simulink model "elec522_sysgen_block_LAB3"  (Simulink 8.9)
settings: Solver=VariableStepAuto  StartTime=0.0  StopTime=30  RelTol=1e-3
libraries: xbsIndex_r4 x41
settings Model: Creator=rl59  LastModifiedBy=rl59
settings DataIOCC: LimitDataPoints=off  SaveFormat=Dataset  SignalLoggingSaveFormat=Dataset
settings OptimizationCC: LifeSpan=auto
settings DebuggingCC: UnderspecifiedInitializationDetection=Simplified  MergeDetectMultiDrivingBlocksExec=error  FcnCallInpInsideContextMsg=error  StateNameClashWarn=none  SFUnexpectedBacktrackingDiag=error  SFNoUnconditionalDefaultTransitionDiag=error  SFExecutionAtInitializationDiag=warning
settings HardwareCC: ProdBitPerPointer=64  ProdBitPerSizeT=64  ProdBitPerPtrDiffT=64  ProdLargestAtomicFloat=Float  ProdIntDivRoundTo=Zero  ProdEndianess=LittleEndian  ProdWordSize=64  ProdHWDeviceType=Intel->x86-64 (Windows64)
settings ModelReferenceCC: PropagateSignalLabelsOutOfModel=on
settings GRTTargetCC: TargetLangStandard=C99 (ISO)  GeneratePreprocessorConditionals=Use local settings  CombineOutputUpdateFcns=on  GRTInterface=off
settings ConfigComp: CovMetricSettings=dwe  CovHtmlReporting=off  CovSaveCumulativeToWorkspaceVar=off  CovSaveSingleToWorkspaceVar=off  CovExternalEMLEnable=on

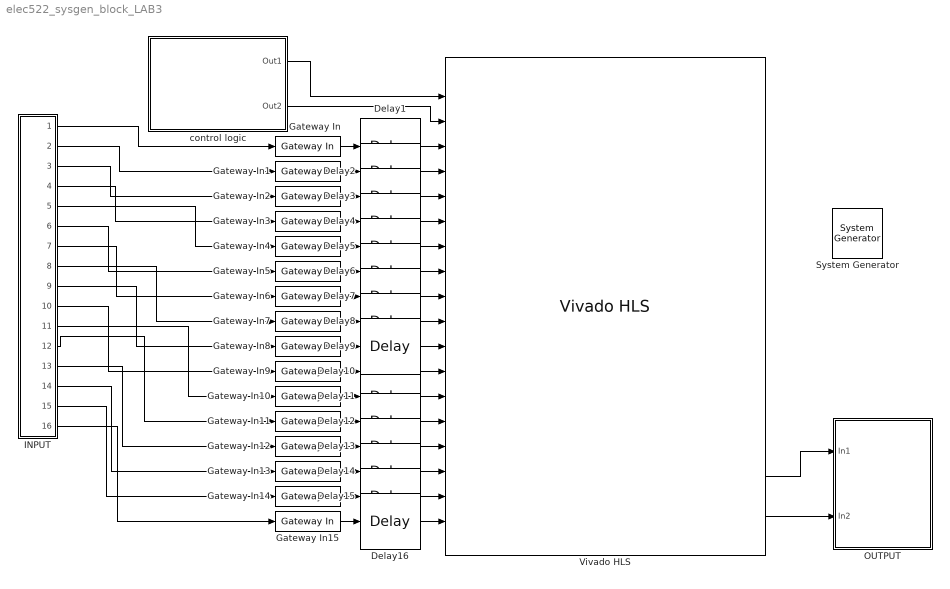
== system elec522_sysgen_block_LAB3 ==
  " System Generator" : xbsIndex_r4/ System Generator  Tag=genX  xilinxfamily=kintex7  part=xc7k325t  speed=-3  package=fbg676  synthesis_tool=Vivado  clock_wrapper=Clock Enables  directory=./netlist  proj_type=Vivado  Synth_file=Vivado Synthesis Defaults  Impl_file=Vivado Implementation Defaults  testbench=off  simulink_period=1  sysclk_period=10  dcm_input_clock_period=10  incr_netlist=off  trim_vbits=Everywhere in SubSystem  dbl_ovrd=According to Block Masks  core_generation=According to Block Masks  run_coregen=off  deprecated_control=off  eval_field=0  block_type=sysgen
  Delay{1..16} (16 alike) : xbsIndex_r4/Delay  rst=off  infoeditControl=Selection of Reset will increase slice count due to use of real FFs and instead of SRLs  en=off  latency=4  reg_retiming=off  dbl_ovrd=off  block_type=delay
  Gateway In{,1..15} (16 alike) : xbsIndex_r4/Gateway In  gui_display_data_type=Fixed-point  arith_type="Signed  (2's comp)"  n_bits=16  bin_pt=0  preci_type=Single  exp_width=8  frac_width=24  rows=1  columns=1  quantization="Round  (unbiased: +/- Inf)"  overflow=Saturate  period=1  UseAsADC=off  ADCChannel='1'  interface=None  automatic_assignment=on  address_offset=hex2dec('00')  intf_name=''  intf_description=''  default_value=0  timing_constraint=None  locs_specified=off  LOCs={}  io_standard={}  inherit_from_input=off  hdl_port=on  dbl_ovrd=off  block_type=gatewayin
  INPUT : Subsystem
  OUTPUT : Subsystem
  Vivado HLS : xbsIndex_r4/Vivado HLS  anytable='C:/Users/rl59/Desktop/ELEC522_project3_RAN.LU_WEIXU.PAN/ELEC522_project3_RAN.LU_WEIXU.PAN/ELEC522_project3/solution6'  fast_sim=off  display_datatype=on  rate_propagation_method=Simulink system period  model_file_path=''  latency=1  block_type=hls
      settings: infoedit=This block allows including C,C++ and SystemC source files in System Generator for DSP designs.
  "control logic " : Subsystem
  wires:
  Gateway In/1 -> Delay1/1
  Delay1/1 -> Vivado HLS/3
  Gateway In1/1 -> Delay2/1
  Delay2/1 -> Vivado HLS/4
  Gateway In2/1 -> Delay3/1
  Delay3/1 -> Vivado HLS/5
  Gateway In3/1 -> Delay4/1
  Delay4/1 -> Vivado HLS/6
  Gateway In4/1 -> Delay5/1
  Delay5/1 -> Vivado HLS/7
  Gateway In5/1 -> Delay6/1
  Delay6/1 -> Vivado HLS/8
  Gateway In6/1 -> Delay7/1
  Delay7/1 -> Vivado HLS/9
  Gateway In7/1 -> Delay8/1
  Delay8/1 -> Vivado HLS/10
  Gateway In8/1 -> Delay9/1
  Delay9/1 -> Vivado HLS/11
  Gateway In9/1 -> Delay10/1
  Delay10/1 -> Vivado HLS/12
  Gateway In10/1 -> Delay11/1
  Delay11/1 -> Vivado HLS/13
  Gateway In11/1 -> Delay12/1
  Delay12/1 -> Vivado HLS/14
  Gateway In12/1 -> Delay13/1
  Delay13/1 -> Vivado HLS/15
  Gateway In13/1 -> Delay14/1
  Delay14/1 -> Vivado HLS/16
  Gateway In14/1 -> Delay15/1
  Delay15/1 -> Vivado HLS/17
  Gateway In15/1 -> Delay16/1
  Delay16/1 -> Vivado HLS/18
  INPUT/1(Out1) -> Gateway In/1
  INPUT/2(Out2) -> Gateway In1/1
  INPUT/3(Out3) -> Gateway In2/1
  INPUT/4(Out4) -> Gateway In3/1
  INPUT/5(Out5) -> Gateway In4/1
  INPUT/6(Out6) -> Gateway In5/1
  INPUT/7(Out7) -> Gateway In6/1
  INPUT/8(Out8) -> Gateway In7/1
  INPUT/9(Out9) -> Gateway In8/1
  INPUT/10(Out10) -> Gateway In9/1
  INPUT/11(Out11) -> Gateway In10/1
  INPUT/12(Out12) -> Gateway In11/1
  INPUT/13(Out13) -> Gateway In12/1
  INPUT/14(Out14) -> Gateway In13/1
  INPUT/15(Out15) -> Gateway In14/1
  INPUT/16(Out16) -> Gateway In15/1
  Vivado HLS/39 -> OUTPUT/1(In1)
  Vivado HLS/43 -> OUTPUT/2(In2)
  "control logic "/1(Out1) -> Vivado HLS/1
  "control logic "/2(Out2) -> Vivado HLS/2

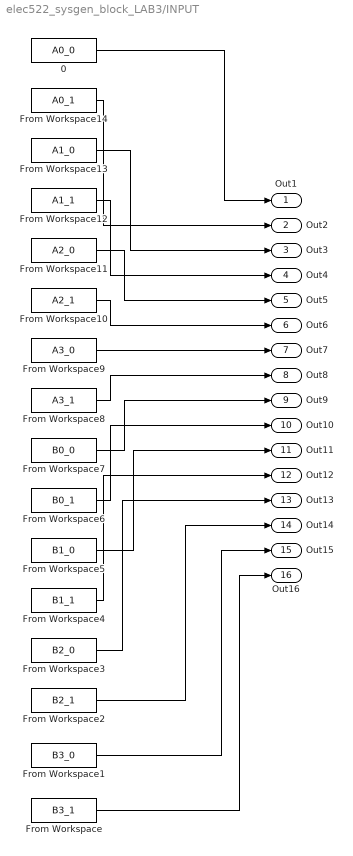
== system elec522_sysgen_block_LAB3/INPUT ==
  0 : FromWorkspace  VariableName=A0_0  SampleTime=1
  From Workspace : FromWorkspace  VariableName=B3_1  SampleTime=1
  From Workspace1 : FromWorkspace  VariableName=B3_0  SampleTime=1
  From Workspace10 : FromWorkspace  VariableName=A2_1  SampleTime=1
  From Workspace11 : FromWorkspace  VariableName=A2_0  SampleTime=1
  From Workspace12 : FromWorkspace  VariableName=A1_1  SampleTime=1
  From Workspace13 : FromWorkspace  VariableName=A1_0  SampleTime=1
  From Workspace14 : FromWorkspace  VariableName=A0_1  SampleTime=1
  From Workspace2 : FromWorkspace  VariableName=B2_1  SampleTime=1
  From Workspace3 : FromWorkspace  VariableName=B2_0  SampleTime=1
  From Workspace4 : FromWorkspace  VariableName=B1_1  SampleTime=1
  From Workspace5 : FromWorkspace  VariableName=B1_0  SampleTime=1
  From Workspace6 : FromWorkspace  VariableName=B0_1  SampleTime=1
  From Workspace7 : FromWorkspace  VariableName=B0_0  SampleTime=1
  From Workspace8 : FromWorkspace  VariableName=A3_1  SampleTime=1
  From Workspace9 : FromWorkspace  VariableName=A3_0  SampleTime=1
  Out1 : Outport
  Out2 : Outport  Port=2
  Out3 : Outport  Port=3
  Out4 : Outport  Port=4
  Out5 : Outport  Port=5
  Out6 : Outport  Port=6
  Out7 : Outport  Port=7
  Out8 : Outport  Port=8
  Out9 : Outport  Port=9
  Out10 : Outport  Port=10
  Out11 : Outport  Port=11
  Out12 : Outport  Port=12
  Out13 : Outport  Port=13
  Out14 : Outport  Port=14
  Out15 : Outport  Port=15
  Out16 : Outport  Port=16
  wires:
  From Workspace3/1 -> Out13/1
  From Workspace2/1 -> Out14/1
  From Workspace13/1 -> Out3/1
  From Workspace7/1 -> Out9/1
  From Workspace5/1 -> Out11/1
  From Workspace1/1 -> Out15/1
  From Workspace14/1 -> Out2/1
  From Workspace4/1 -> Out12/1
  From Workspace10/1 -> Out6/1
  From Workspace11/1 -> Out5/1
  0/1 -> Out1/1
  From Workspace6/1 -> Out10/1
  From Workspace12/1 -> Out4/1
  From Workspace/1 -> Out16/1
  From Workspace9/1 -> Out7/1
  From Workspace8/1 -> Out8/1

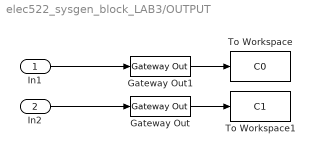
== system elec522_sysgen_block_LAB3/OUTPUT ==
  In1 : Inport
  In2 : Inport  Port=2
  Gateway Out : xbsIndex_r4/Gateway Out  inherit_from_input=off  hdl_port=on  rows=1  columns=1  UseAsDAC=off  DACChannel='1'  interface=None  automatic_assignment=on  address_offset=hex2dec('00')  intf_name=''  intf_description=''  timing_constraint=None  locs_specified=off  LOCs={}  io_standard={}  block_type=gatewayout
  Gateway Out1 : xbsIndex_r4/Gateway Out  inherit_from_input=off  hdl_port=on  rows=1  columns=1  UseAsDAC=off  DACChannel='1'  interface=None  automatic_assignment=on  address_offset=hex2dec('00')  intf_name=''  intf_description=''  timing_constraint=None  locs_specified=off  LOCs={}  io_standard={}  block_type=gatewayout
  To Workspace : ToWorkspace  VariableName=C0  SampleTime=-1
  To Workspace1 : ToWorkspace  VariableName=C1  SampleTime=-1
  wires:
  In2/1 -> Gateway Out/1
  In1/1 -> Gateway Out1/1
  Gateway Out/1 -> To Workspace1/1
  Gateway Out1/1 -> To Workspace/1

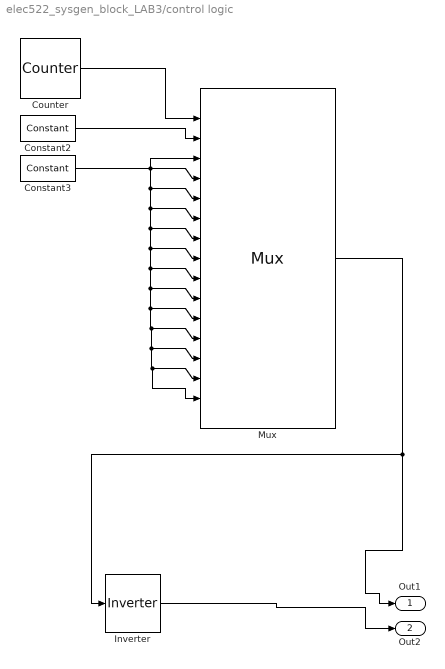
== system elec522_sysgen_block_LAB3/control logic  ==
  Constant2 : xbsIndex_r4/Constant  const=1.0  gui_display_data_type=Boolean  arith_type=Boolean  n_bits=16  bin_pt=14  preci_type=Single  exp_width=8  frac_width=24  explicit_period=on  period=1  equ=P=C  opselect=C  inp2=PCIN>>17  opr=+  inp1=P  carry=CIN  dbl_ovrd=off  block_type=constant
  Constant3 : xbsIndex_r4/Constant  const=0  gui_display_data_type=Boolean  arith_type=Boolean  n_bits=16  bin_pt=14  preci_type=Single  exp_width=8  frac_width=24  explicit_period=on  period=1  equ=P=C  opselect=C  inp2=PCIN>>17  opr=+  inp1=P  carry=CIN  dbl_ovrd=off  block_type=constant
  Counter : xbsIndex_r4/Counter  cnt_type=Count Limited  cnt_to=13  operation=Up  start_count=0  cnt_by_val=1  arith_type=Unsigned  n_bits=4  bin_pt=0  load_pin=off  rst=off  en=off  explicit_period=on  period=1  use_behavioral_HDL=off  implementation=Fabric  dbl_ovrd=off  block_type=counter
  Inverter : xbsIndex_r4/Inverter  en=off  latency=1  dbl_ovrd=off  block_type=inv
  Mux : xbsIndex_r4/Mux  inputs=14  en=off  latency=0  precision=Full  arith_type=Unsigned  n_bits=16  bin_pt=14  quantization=Truncate  overflow=Wrap  dbl_ovrd=off  block_type=mux
  Out1 : Outport
  Out2 : Outport  Port=2
  wires:
  Constant2/1 -> Mux/2
  Constant3/1 -> Mux/15, Mux/14, Mux/13, Mux/12, Mux/11, Mux/10, Mux/9, Mux/8, Mux/7, Mux/6, Mux/5, Mux/3, Mux/4
  Counter/1 -> Mux/1
  Mux/1 -> Out1/1, Inverter/1
  Inverter/1 -> Out2/1
